simulink model "VITM_sfun"  (R2024b)
settings: Solver=FixedStepDiscrete  StartTime=0.0  StopTime=inf  RelTol=1e-3  EnableMultiTasking=on
values from neighbouring files (symbols this model uses):
  vitc_CellPackVolTol = 12    [VITM_init.m]
  vitc_CellTempFaultTimer = 10    [VITM_init.m]
  vitc_CellTempFilterC = 1.0    (= 1)    [VITM_init.m]
  vitc_CellTempHighFaultReset = 0    [VITM_init.m]
  vitc_CellTempLowFaultReset = 0    [VITM_init.m]
  vitc_CellTempMax = 70    [VITM_init.m]
  vitc_CellTempMin = -40    [VITM_init.m]
  vitc_CellVolFilterC = 1    [VITM_init.m]
  vitc_CellVoltageFaultTimer = 2    [VITM_init.m]
  vitc_CellVoltageHighFaultReset = 0    [VITM_init.m]
  vitc_CellVoltageLowFaultReset = 0    [VITM_init.m]
  vitc_CellVoltageMax = 4.2    [VITM_init.m]
  vitc_CellVoltageMin = 2.7    [VITM_init.m]
  vitc_CoolantInletTFaultReset = 0    [VITM_init.m]
  vitc_CoolantInletTLowerLim = -40    [VITM_init.m]
  vitc_CoolantInletTUpperLim = 70    [VITM_init.m]
  vitc_CoolantOutletTFaultReset = 0    [VITM_init.m]
  vitc_CoolantOutletTLowerLim = -40    [VITM_init.m]
  vitc_CoolantOutletTUpperLim = 70    [VITM_init.m]
  vitc_CoolantTempFaultCounter = 5    [VITM_init.m]
  vitc_CoolantTFilterC = 0.9    [VITM_init.m]
  vitc_HVILFaultCounter = 1    [VITM_init.m]
  vitc_HVILFaultReset = 0    [VITM_init.m]
  vitc_PackCurFilterC = 1    [VITM_init.m]
  vitc_PackCurrentFaultReset = 0    [VITM_init.m]
  vitc_PackCurrentFaultTimer = 1    [VITM_init.m]
  vitc_PackCurrentLimit = 300    [VITM_init.m]
  vitc_PackVolFilterC = 1    [VITM_init.m]
  vitc_PackVoltageFaultReset = 0    [VITM_init.m]
  vitc_PackVoltageFaultTimer = 10    [VITM_init.m]
  vitc_VehVolFilterC = 1    [VITM_init.m]
  vitk_NumberInPara = 1    [VITM_init.m]
  vitk_NumberInSeries = 40    [VITM_init.m]
  vitk_stepSize = 0.1    [VITM_init.m]
settings Model: TunableVars=vitc_CellPackVolTol,vitc_CellTempFaultTimer,vitc_CellTempFilterC,vitc_CellTempHighFaultReset,vitc_CellTempLowFaultReset,vitc_CellTempMax,vitc_CellTempMin,vitc_CellVolFilterC,vitc_CellVoltageFaultTimer,vitc_CellVoltageHighFaultReset,vitc_CellVoltageLowFaultReset,vitc_CellVoltageMax,vitc_CellVoltageMin,vitc_CoolantInletTFaultReset,vitc_CoolantInletTLowerLim,vitc_CoolantInletTUpperLim,vitc_CoolantOutletTFaultReset,vitc_CoolantOutletTLowerLim,vitc_CoolantOutletTUpperLim,vitc_CoolantTFilterC,vitc_CoolantTempFaultCounter,vitc_HVILFaultCounter,vitc_HVILFaultReset,vitc_PackCurFilterC,vitc_PackCurrentFaultReset,vitc_PackCurrentFaultTimer,vitc_PackCurrentLimit,vitc_PackVolFilterC,vitc_PackVoltageFaultReset,vitc_PackVoltageFaultTimer,vitc_VehVolFilterC,vitk_NumberInPara,vitk_NumberInSeries,vitk_stepSize  TunableVarsStorageClass=Auto,Auto,Auto,Auto,Auto,Auto,Auto,Auto,Auto,Auto,Auto,Auto,Auto,Auto,Auto,Auto,Auto,Auto,Auto,Auto,Auto,Auto,Auto,Auto,Auto,Auto,Auto,Auto,Auto,Auto,Auto,Auto,Auto,Auto  TunableVarsTypeQualifier=,,,,,,,,,,,,,,,,,,,,,,,,,,,,,,,,,  Creator=nctzv8  LastModifiedBy=voillat
settings ConfigSet: Description=OpenECU configuration set for code generation under RTW-EC.
settings SolverCC: AlgebraicLoopSolver=TrustRegion  PositivePriorityOrder=on
settings DataIOCC: LimitDataPoints=on  SaveFormat=Array  SignalLoggingSaveFormat=ModelDataLogs
settings OptimizationCC: DefaultParameterBehavior=Inlined  InlineInvariantSignals=on  ExpressionDepthLimit=2147483647  StateBitsets=on  DataBitsets=on  ZeroExternalMemoryAtStartup=off  ZeroInternalMemoryAtStartup=off  NoFixptDivByZeroProtection=on  EfficientFloat2IntCast=on  LifeSpan=1  EfficientTunableParamExpr=on
settings DebuggingCC: SaveWithParameterizedLinksMsg=none  SignalResolutionControl=TryResolveAllWithWarning  MultiTaskDSMMsg=warning  MultiTaskCondExecSysMsg=none  SingleTaskRateTransMsg=error  CheckMatrixSingularityMsg=warning  VectorMatrixConversionMsg=warning  SignalLabelMismatchMsg=warning  UnconnectedInputMsg=warning  UnconnectedOutputMsg=warning  UnconnectedLineMsg=warning  AllowSymbolicDim=off  StateNameClashWarn=warning  SFUnexpectedBacktrackingDiag=warning  SFNoUnconditionalDefaultTransitionDiag=warning  SFExecutionAtInitializationDiag=none  ArithmeticOperatorsInVariantConditions=warning
settings HardwareCC: ProdBitPerPointer=32  ProdBitPerSizeT=32  ProdBitPerPtrDiffT=32  ProdLargestAtomicInteger=Long  ProdLargestAtomicFloat=Double  ProdEndianess=BigEndian  ProdWordSize=32  ProdHWDeviceType=Freescale->32-bit PowerPC  TargetIntDivRoundTo=Zero  TargetEndianess=BigEndian  TargetHWDeviceType=Freescale->32-bit PowerPC  ProdEqTarget=off
settings ModelReferenceCC: EnableRefExpFcnMdlSchedulingChecks=on  PropagateSignalLabelsOutOfModel=off
settings SFSimCC: SimUseLocalCustomCode=off  MATLABDynamicMemAlloc=off  CustomCodeUndefinedFunction=UseInterfaceOnly
settings RTWCC: Description=OpenECU Platform Target (ERT, optimised floating-point code)  SystemTargetFile=openecu_ert.tlc  MakeCommand=make_rtw optimized_floating_point=1  TemplateMakefile=openecu_ert_r2015b_64.tmf  RetainRTWFile=on  RTWUseLocalCustomCode=off  IncludeHyperlinkInReport=on  GPUComputeCapability=3.5
settings CodeAppCC: ForceParamTrailComments=on  IgnoreCustomStorageClasses=off  SimulinkDataObjDesc=on  CustomSymbolStrType=$N$R$M  InsertBlockDesc=on  StateflowObjectComments=on  InternalIdentifier=Classic
settings STFCustomTargetCC: TargetLibSuffix=.a  GenerateSampleERTMain=on  IncludeMdlTerminateFcn=off  CombineOutputUpdateFcns=on  IncludeFileDelimiter=UseQuote  ERTCustomFileBanners=on  SupportContinuousTime=off  RemoveResetFunc=on  MATLABClassNameForMDSCustomization=Simulink.SoftwareTarget.ERTCustomization  SystemTargetFile=openecu_ert.tlc
settings ERTTargetCC: MultiwordLength=2048  GenerateSampleERTMain=on  ParMdlRefBuildCompliant=off  CompOptLevelCompliant=off  ConcurrentExecutionCompliant=off  IncludeMdlTerminateFcn=off  IncludeFileDelimiter=UseQuote  SupportNonInlinedSFcns=on  ModelStepFunctionPrototypeControlCompliant=off  CPPClassGenCompliant=off  UseToolchainInfoCompliant=off  ExtModeMexFile=noextcomm  ERTSrcFileBannerTemplate=oe_code_c_template.cgt  ERTHdrFileBannerTemplate=oe_code_h_template.cgt  ERTDataSrcFileTemplate=oe_data_c_template.cgt  ERTDataHdrFileTemplate=oe_data_h_template.cgt  ERTCustomFileTemplate=example_file_process.tlc  GlobalDataDefinition=InSeparateSourceFile  GlobalDataReference=InSeparateHeaderFile  ConvertIfToSwitch=off  SuppressUnreachableDefaultCases=off  EnableUserReplacementTypes=on  DynamicArrayContainerType=coder::array
settings ConfigComp: CovMetricSettings=dw  CovSaveCumulativeToWorkspaceVar=on  CovSaveSingleToWorkspaceVar=on  CovExternalEMLEnable=off

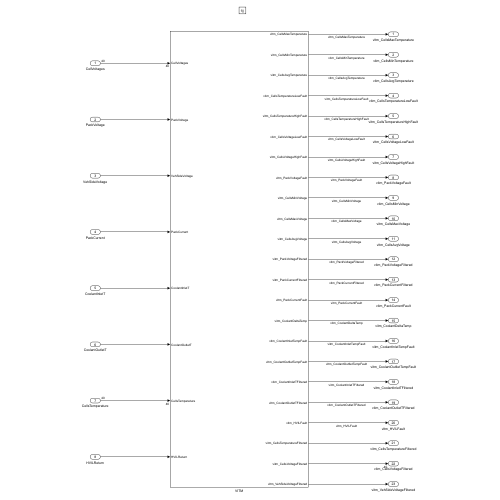
[thumbnail: Simulink's stored preview of the top-level diagram]
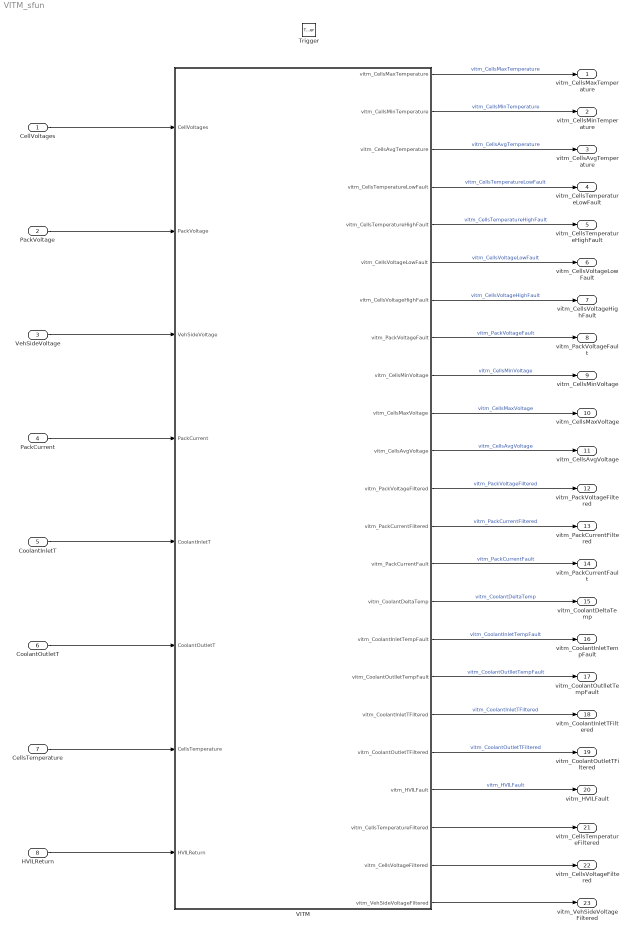
== system VITM_sfun ==
  CellVoltages : Inport  PortDimensions=40
  PackVoltage : Inport  Port=2
  VehSideVoltage : Inport  Port=3
  PackCurrent : Inport  Port=4
  CoolantInletT : Inport  Port=5
  CoolantOutletT : Inport  Port=6
  CellsTemperature : Inport  Port=7  PortDimensions=40
  HVILReturn : Inport  Port=8
  Trigger : TriggerPort  TriggerType=function-call  VariantControl=(inherit)  PortDimensions=1
  VITM : Subsystem  mask{prm_to_disp=[1..10], sfcnParam1=vitc_CellPackVolTol, sfcnParam2=vitc_CellTempFaultTimer, sfcnParam3=vitc_CellTempFilterC, sfcnParam4=vitc_CellTempHighFaultReset, sfcnParam5=vitc_CellTempLowFaultReset, sfcnParam6=vitc_CellTempMax, sfcnParam7=vitc_CellTempMin, sfcnParam8=vitc_CellVolFilterC, sfcnParam9=vitc_CellVoltageFaultTimer, sfcnParam10=vitc_CellVoltageHighFaultReset, sfcnParam11=vitc_CellVoltageLowFaultReset, sfcnParam12=vitc_CellVoltageMax, sfcnParam13=vitc_CellVoltageMin, sfcnParam14=vitc_CoolantInletTFaultReset, sfcnParam15=vitc_CoolantInletTLowerLim, sfcnParam16=vitc_CoolantInletTUpperLim, sfcnParam17=vitc_CoolantOutletTFaultReset, sfcnParam18=vitc_CoolantOutletTLowerLim, sfcnParam19=vitc_CoolantOutletTUpperLim, sfcnParam20=vitc_CoolantTFilterC, sfcnParam21=vitc_CoolantTempFaultCounter, sfcnParam22=vitc_HVILFaultCounter, sfcnParam23=vitc_HVILFaultReset, sfcnParam24=vitc_PackCurFilterC, sfcnParam25=vitc_PackCurrentFaultReset, sfcnParam26=vitc_PackCurrentFaultTimer, sfcnParam27=vitc_PackCurrentLimit, sfcnParam28=vitc_PackVolFilterC, sfcnParam29=vitc_PackVoltageFaultReset, sfcnParam30=vitc_PackVoltageFaultTimer, sfcnParam31=vitc_VehVolFilterC, sfcnParam32=vitk_NumberInPara, sfcnParam33=vitk_NumberInSeries, sfcnParam34=vitk_stepSize}
      mask prompts: prm_to_disp "Display S-function Parameters:"; sfcnParam1 "vitc_CellPackVolTol:"; sfcnParam2 "vitc_CellTempFaultTimer:"; sfcnParam3 "vitc_CellTempFilterC:"; sfcnParam4 "vitc_CellTempHighFaultReset:"; sfcnParam5 "vitc_CellTempLowFaultReset:"; sfcnParam6 "vitc_CellTempMax:"; sfcnParam7 "vitc_CellTempMin:"; sfcnParam8 "vitc_CellVolFilterC:"; sfcnParam9 "vitc_CellVoltageFaultTimer:"; sfcnParam10 "vitc_CellVoltageHighFaultReset:"; sfcnParam11 "vitc_CellVoltageLowFaultReset:"; sfcnParam12 "vitc_CellVoltageMax:"; sfcnParam13 "vitc_CellVoltageMin:"; sfcnParam14 "vitc_CoolantInletTFaultReset:"; sfcnParam15 "vitc_CoolantInletTLowerLim:"; sfcnParam16 "vitc_CoolantInletTUpperLim:"; sfcnParam17 "vitc_CoolantOutletTFaultReset:"; sfcnParam18 "vitc_CoolantOutletTLowerLim:"; sfcnParam19 "vitc_CoolantOutletTUpperLim:"; sfcnParam20 "vitc_CoolantTFilterC:"; sfcnParam21 "vitc_CoolantTempFaultCounter:"; sfcnParam22 "vitc_HVILFaultCounter:"; sfcnParam23 "vitc_HVILFaultReset:"; sfcnParam24 "vitc_PackCurFilterC:"; sfcnParam25 "vitc_PackCurrentFaultReset:"; sfcnParam26 "vitc_PackCurrentFaultTimer:"; sfcnParam27 "vitc_PackCurrentLimit:"; sfcnParam28 "vitc_PackVolFilterC:"; sfcnParam29 "vitc_PackVoltageFaultReset:"; sfcnParam30 "vitc_PackVoltageFaultTimer:"; sfcnParam31 "vitc_VehVolFilterC:"; sfcnParam32 "vitk_NumberInPara:"; sfcnParam33 "vitk_NumberInSeries:"; sfcnParam34 "vitk_stepSize:"
      mask help: Simulink:masks:GenSFuncDesc_MD
      mask Help: eval('feval(''rtwprivate'',''rtwhelpview'',''rtw_sfcn_block'')');
      mask TypeOptions prm_to_disp: [1..10] | [11..20] | [21..30] | [31..34]
      mask Callback prm_to_disp: slmaskprmdispcntrl(gcbh)
  vitm_CellsMaxTemperature : Outport
  vitm_CellsMinTemperature : Outport  Port=2
  vitm_CellsAvgTemperature : Outport  Port=3
  vitm_CellsTemperatureLowFault : Outport  Port=4
  vitm_CellsTemperatureHighFault : Outport  Port=5
  vitm_CellsVoltageLowFault : Outport  Port=6
  vitm_CellsVoltageHighFault : Outport  Port=7
  vitm_PackVoltageFault : Outport  Port=8
  vitm_CellsMinVoltage : Outport  Port=9
  vitm_CellsMaxVoltage : Outport  Port=10
  vitm_CellsAvgVoltage : Outport  Port=11
  vitm_PackVoltageFiltered : Outport  Port=12
  vitm_PackCurrentFiltered : Outport  Port=13
  vitm_PackCurrentFault : Outport  Port=14
  vitm_CoolantDeltaTemp : Outport  Port=15
  vitm_CoolantInletTempFault : Outport  Port=16
  vitm_CoolantOutlletTempFault : Outport  Port=17
  vitm_CoolantInletTFiltered : Outport  Port=18
  vitm_CoolantOutletTFiltered : Outport  Port=19
  vitm_HVILFault : Outport  Port=20
  vitm_CellsTemperatureFiltered : Outport  Port=21
  vitm_CellsVoltageFiltered : Outport  Port=22  PortDimensions=40
  vitm_VehSideVoltageFiltered : Outport  Port=23
  wires:
  CellVoltages/1 -> VITM/1(CellVoltages)
  PackVoltage/1 -> VITM/2(PackVoltage)
  VehSideVoltage/1 -> VITM/3(VehSideVoltage)
  PackCurrent/1 -> VITM/4(PackCurrent)
  CoolantInletT/1 -> VITM/5(CoolantInletT)
  CoolantOutletT/1 -> VITM/6(CoolantOutletT)
  CellsTemperature/1 -> VITM/7(CellsTemperature)
  HVILReturn/1 -> VITM/8(HVILReturn)
  VITM/2(vitm_CellsMinTemperature) -> vitm_CellsMinTemperature/1  "vitm_CellsMinTemperature"
  VITM/3(vitm_CellsAvgTemperature) -> vitm_CellsAvgTemperature/1  "vitm_CellsAvgTemperature"
  VITM/1(vitm_CellsMaxTemperature) -> vitm_CellsMaxTemperature/1  "vitm_CellsMaxTemperature"
  VITM/4(vitm_CellsTemperatureLowFault) -> vitm_CellsTemperatureLowFault/1  "vitm_CellsTemperatureLowFault"
  VITM/6(vitm_CellsVoltageLowFault) -> vitm_CellsVoltageLowFault/1  "vitm_CellsVoltageLowFault"
  VITM/7(vitm_CellsVoltageHighFault) -> vitm_CellsVoltageHighFault/1  "vitm_CellsVoltageHighFault"
  VITM/5(vitm_CellsTemperatureHighFault) -> vitm_CellsTemperatureHighFault/1  "vitm_CellsTemperatureHighFault"
  VITM/9(vitm_CellsMinVoltage) -> vitm_CellsMinVoltage/1  "vitm_CellsMinVoltage"
  VITM/8(vitm_PackVoltageFault) -> vitm_PackVoltageFault/1  "vitm_PackVoltageFault"
  VITM/18(vitm_CoolantInletTFiltered) -> vitm_CoolantInletTFiltered/1  "vitm_CoolantInletTFiltered"
  VITM/10(vitm_CellsMaxVoltage) -> vitm_CellsMaxVoltage/1  "vitm_CellsMaxVoltage"
  VITM/12(vitm_PackVoltageFiltered) -> vitm_PackVoltageFiltered/1  "vitm_PackVoltageFiltered"
  VITM/14(vitm_PackCurrentFault) -> vitm_PackCurrentFault/1  "vitm_PackCurrentFault"
  VITM/15(vitm_CoolantDeltaTemp) -> vitm_CoolantDeltaTemp/1  "vitm_CoolantDeltaTemp"
  VITM/13(vitm_PackCurrentFiltered) -> vitm_PackCurrentFiltered/1  "vitm_PackCurrentFiltered"
  VITM/11(vitm_CellsAvgVoltage) -> vitm_CellsAvgVoltage/1  "vitm_CellsAvgVoltage"
  VITM/16(vitm_CoolantInletTempFault) -> vitm_CoolantInletTempFault/1  "vitm_CoolantInletTempFault"
  VITM/17(vitm_CoolantOutlletTempFault) -> vitm_CoolantOutlletTempFault/1  "vitm_CoolantOutlletTempFault"
  VITM/19(vitm_CoolantOutletTFiltered) -> vitm_CoolantOutletTFiltered/1  "vitm_CoolantOutletTFiltered"
  VITM/23(vitm_VehSideVoltageFiltered) -> vitm_VehSideVoltageFiltered/1
  VITM/22(vitm_CellsVoltageFiltered) -> vitm_CellsVoltageFiltered/1
  VITM/21(vitm_CellsTemperatureFiltered) -> vitm_CellsTemperatureFiltered/1
  VITM/20(vitm_HVILFault) -> vitm_HVILFault/1  "vitm_HVILFault"

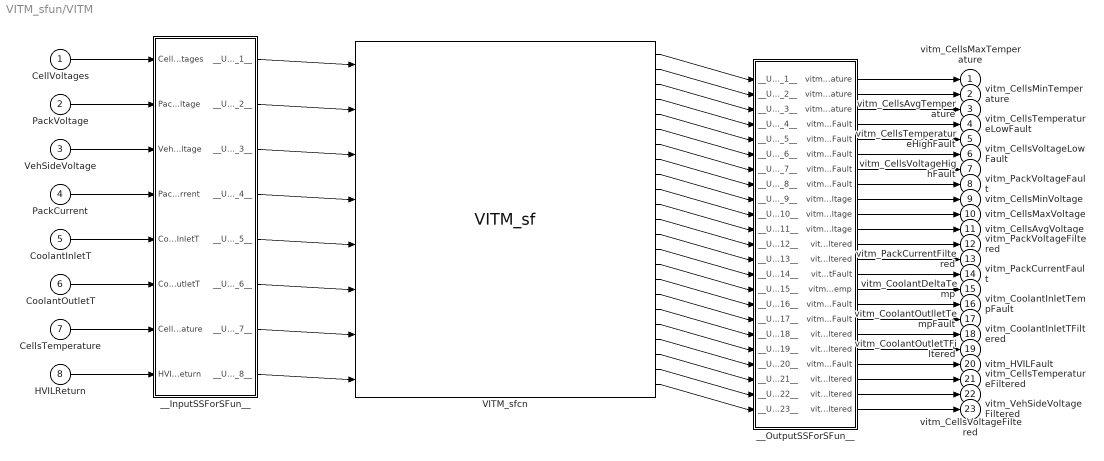
== system VITM_sfun/VITM ==
  CellVoltages : Inport  PortDimensions=40
  PackVoltage : Inport  Port=2
  VehSideVoltage : Inport  Port=3
  PackCurrent : Inport  Port=4
  CoolantInletT : Inport  Port=5
  CoolantOutletT : Inport  Port=6
  CellsTemperature : Inport  Port=7  PortDimensions=40
  HVILReturn : Inport  Port=8
  VITM_sfcn : S-Function  FunctionName=VITM_sf  Parameters=sfcnParam1, sfcnParam2, sfcnParam3, sfcnParam4, sfcnParam5, sfcnParam6, sfcnParam7, sfcnParam8, sfcnParam9, sfcnParam10, sfcnParam11, sfcnParam12, sfcnParam13, sfcnParam14, sfcnParam15, sfcnParam16, sfcnParam17, sfcnParam18, sfcnParam19, sfcnParam20, sfcnParam21, sfcnParam22, sfcnParam23, sfcnParam24, sfcnParam25, sfcnParam26, sfcnParam27, sfcnParam28, sfcnParam29, sfcnParam30, sfcnParam31, sfcnParam32, sfcnParam33, sfcnParam34  SFunctionModules=""  SFunctionDeploymentMode=off  EnableBusSupport=off  mask{rtw_sf_name=VITM_sf, showVar=off, prm_to_disp=[1..10], sfcnParam1=sfcnParam1, sfcnParam2=sfcnParam2, sfcnParam3=sfcnParam3, sfcnParam4=sfcnParam4, sfcnParam5=sfcnParam5, sfcnParam6=sfcnParam6, sfcnParam7=sfcnParam7, sfcnParam8=sfcnParam8, sfcnParam9=sfcnParam9, sfcnParam10=sfcnParam10, sfcnParam11=sfcnParam11, sfcnParam12=sfcnParam12, sfcnParam13=sfcnParam13, sfcnParam14=sfcnParam14, sfcnParam15=sfcnParam15, sfcnParam16=sfcnParam16, sfcnParam17=sfcnParam17, sfcnParam18=sfcnParam18, sfcnParam19=sfcnParam19, sfcnParam20=sfcnParam20, sfcnParam21=sfcnParam21, sfcnParam22=sfcnParam22, sfcnParam23=sfcnParam23, sfcnParam24=sfcnParam24, sfcnParam25=sfcnParam25, sfcnParam26=sfcnParam26, sfcnParam27=sfcnParam27, sfcnParam28=sfcnParam28, sfcnParam29=sfcnParam29, sfcnParam30=sfcnParam30, sfcnParam31=sfcnParam31, sfcnParam32=sfcnParam32, sfcnParam33=sfcnParam33, sfcnParam34=sfcnParam34}
      mask prompts: rtw_sf_name "Simulink:masks:GenSFuncName_MP"; showVar "Simulink:masks:GenSFuncShowModuleList_MP"; prm_to_disp "Display S-function Parameters:"; sfcnParam1 "vitc_CellPackVolTol:"; sfcnParam2 "vitc_CellTempFaultTimer:"; sfcnParam3 "vitc_CellTempFilterC:"; sfcnParam4 "vitc_CellTempHighFaultReset:"; sfcnParam5 "vitc_CellTempLowFaultReset:"; sfcnParam6 "vitc_CellTempMax:"; sfcnParam7 "vitc_CellTempMin:"; sfcnParam8 "vitc_CellVolFilterC:"; sfcnParam9 "vitc_CellVoltageFaultTimer:"; sfcnParam10 "vitc_CellVoltageHighFaultReset:"; sfcnParam11 "vitc_CellVoltageLowFaultReset:"; sfcnParam12 "vitc_CellVoltageMax:"; sfcnParam13 "vitc_CellVoltageMin:"; sfcnParam14 "vitc_CoolantInletTFaultReset:"; sfcnParam15 "vitc_CoolantInletTLowerLim:"; sfcnParam16 "vitc_CoolantInletTUpperLim:"; sfcnParam17 "vitc_CoolantOutletTFaultReset:"; sfcnParam18 "vitc_CoolantOutletTLowerLim:"; sfcnParam19 "vitc_CoolantOutletTUpperLim:"; sfcnParam20 "vitc_CoolantTFilterC:"; sfcnParam21 "vitc_CoolantTempFaultCounter:"; sfcnParam22 "vitc_HVILFaultCounter:"; sfcnParam23 "vitc_HVILFaultReset:"; sfcnParam24 "vitc_PackCurFilterC:"; sfcnParam25 "vitc_PackCurrentFaultReset:"; sfcnParam26 "vitc_PackCurrentFaultTimer:"; sfcnParam27 "vitc_PackCurrentLimit:"; sfcnParam28 "vitc_PackVolFilterC:"; sfcnParam29 "vitc_PackVoltageFaultReset:"; sfcnParam30 "vitc_PackVoltageFaultTimer:"; sfcnParam31 "vitc_VehVolFilterC:"; sfcnParam32 "vitk_NumberInPara:"; sfcnParam33 "vitk_NumberInSeries:"; sfcnParam34 "vitk_stepSize:"
      mask help: Simulink:masks:GenSFuncDesc_MD
      mask init:
      | displist = '';
      | if ~strcmp(get_param(gcb, 'FunctionName'), rtw_sf_name);
      |   set_param(gcb, 'FunctionName', rtw_sf_name);
      | end
      | % Check if we are generating code
      | rtw_mode = false;
      | if strcmpi(get_param(bdroot(gcb),'SimulationStatus'),'Initializing')
      | 	rtw_mode = strcmpi(get_param(bdroot(gcb),'BuildingRTWCode'),'on') && ...
      | 		~strcmpi(get_param(bdroot(gcb),'TargetStyle'),'SimulationTarget');
      | end
      | if showVar || rtw_mode
      | 	if exist('rtwsfunc') == 2 | exist('rtwsfunc') == 6
      | 		tmplist = rtwsfunc(rtw_sf_name,gcb);
      | 		tmplist = DAStudio.message('Simulink:masks:GenSFuncListOfModules_IC', tmplist);
      | 	elseif showVar
      | 		tmplist1 = DAStudio.message('Simulink:masks:GenSFuncListOfModules_IC', '');
      |         tmplist2 = DAStudio.message('Simulink:masks:GenSFuncNotLicensed_IC');
      |         tmplist = [tmplist1 tmplist2];
      |  	end
      | end
      | if showVar
      |   displist = tmplist;
      | end
      settings: CopyFcn=|
      | if ~strcmp(get_param(gcb,'Linkstatus'),'none') && ...
      | ~strcmp(get_param(gcb,'Linkstatus'),'implicit')
      |   set_param(gcb,'LinkStatus','none');
      | end
      mask Help: eval('feval(''rtwprivate'',''rtwhelpview'',''rtw_sfcn_block'')');
      mask TypeOptions prm_to_disp: [1..10] | [11..20] | [21..30] | [31..34]
      mask Callback prm_to_disp: slmaskprmdispcntrl(gcbh)
      mask Display:
      | port_label('input',1,'CellVoltages');
      | port_label('input',2,'PackVoltage');
      | port_label('input',3,'VehSideVoltage');
      | port_label('input',4,'PackCurrent');
      | port_label('input',5,'CoolantInletT');
      | port_label('input',6,'CoolantOutletT');
      | port_label('input',7,'CellsTemperature');
      | port_label('input',8,'HVILReturn');
      | port_label('output',1,'vitm_CellsMaxTemperature');
      | port_label('output',2,'vitm_CellsMinTemperature');
      | port_label('output',3,'vitm_CellsAvgTemperature');
      | port_label('output',4,'vitm_CellsTemperatureLowFault');
      | port_label('output',5,'vitm_CellsTemperatureHighFault');
      | port_label('output',6,'vitm_CellsVoltageLowFault');
      | port_label('output',7,'vitm_CellsVoltageHighFault');
      | port_label('output',8,'vitm_PackVoltageFault');
      | port_label('output',9,'vitm_CellsMinVoltage');
      | port_label('output',10,'vitm_CellsMaxVoltage');
      | port_label('output',11,'vitm_CellsAvgVoltage');
      | port_label('output',12,'vitm_PackVoltageFiltered');
      | port_label('output',13,'vitm_PackCurrentFiltered');
      | port_label('output',14,'vitm_PackCurrentFault');
      | port_label('output',15,'vitm_CoolantDeltaTemp');
      | port_label('output',16,'vitm_CoolantInletTempFault');
      | port_label('output',17,'vitm_CoolantOutlletTempFault');
      | port_label('output',18,'vitm_CoolantInletTFiltered');
      | port_label('output',19,'vitm_CoolantOutletTFiltered');
      | port_label('output',20,'vitm_HVILFault');
      | port_label('output',21,'vitm_CellsTemperatureFiltered');
      | port_label('output',22,'vitm_CellsVoltageFiltered');
      | port_label('output',23,'vitm_VehSideVoltageFiltered');
  __InputSSForSFun__ : Subsystem
  __OutputSSForSFun__ : Subsystem
  vitm_CellsMaxTemperature : Outport
  vitm_CellsMinTemperature : Outport  Port=2
  vitm_CellsAvgTemperature : Outport  Port=3
  vitm_CellsTemperatureLowFault : Outport  Port=4
  vitm_CellsTemperatureHighFault : Outport  Port=5
  vitm_CellsVoltageLowFault : Outport  Port=6
  vitm_CellsVoltageHighFault : Outport  Port=7
  vitm_PackVoltageFault : Outport  Port=8
  vitm_CellsMinVoltage : Outport  Port=9
  vitm_CellsMaxVoltage : Outport  Port=10
  vitm_CellsAvgVoltage : Outport  Port=11
  vitm_PackVoltageFiltered : Outport  Port=12
  vitm_PackCurrentFiltered : Outport  Port=13
  vitm_PackCurrentFault : Outport  Port=14
  vitm_CoolantDeltaTemp : Outport  Port=15
  vitm_CoolantInletTempFault : Outport  Port=16
  vitm_CoolantOutlletTempFault : Outport  Port=17
  vitm_CoolantInletTFiltered : Outport  Port=18
  vitm_CoolantOutletTFiltered : Outport  Port=19
  vitm_HVILFault : Outport  Port=20
  vitm_CellsTemperatureFiltered : Outport  Port=21
  vitm_CellsVoltageFiltered : Outport  Port=22
  vitm_VehSideVoltageFiltered : Outport  Port=23
  wires:
  CellVoltages/1 -> __InputSSForSFun__/1(CellVoltages)
  PackVoltage/1 -> __InputSSForSFun__/2(PackVoltage)
  VehSideVoltage/1 -> __InputSSForSFun__/3(VehSideVoltage)
  PackCurrent/1 -> __InputSSForSFun__/4(PackCurrent)
  CoolantInletT/1 -> __InputSSForSFun__/5(CoolantInletT)
  CoolantOutletT/1 -> __InputSSForSFun__/6(CoolantOutletT)
  CellsTemperature/1 -> __InputSSForSFun__/7(CellsTemperature)
  HVILReturn/1 -> __InputSSForSFun__/8(HVILReturn)
  __InputSSForSFun__/1(__UniqueOutportName__1__) -> VITM_sfcn/1
  __InputSSForSFun__/2(__UniqueOutportName__2__) -> VITM_sfcn/2
  __InputSSForSFun__/3(__UniqueOutportName__3__) -> VITM_sfcn/3
  __InputSSForSFun__/4(__UniqueOutportName__4__) -> VITM_sfcn/4
  __InputSSForSFun__/5(__UniqueOutportName__5__) -> VITM_sfcn/5
  __InputSSForSFun__/6(__UniqueOutportName__6__) -> VITM_sfcn/6
  __InputSSForSFun__/7(__UniqueOutportName__7__) -> VITM_sfcn/7
  __InputSSForSFun__/8(__UniqueOutportName__8__) -> VITM_sfcn/8
  VITM_sfcn/1 -> __OutputSSForSFun__/1(__UniqueInportName__1__)
  VITM_sfcn/2 -> __OutputSSForSFun__/2(__UniqueInportName__2__)
  VITM_sfcn/3 -> __OutputSSForSFun__/3(__UniqueInportName__3__)
  VITM_sfcn/4 -> __OutputSSForSFun__/4(__UniqueInportName__4__)
  VITM_sfcn/5 -> __OutputSSForSFun__/5(__UniqueInportName__5__)
  VITM_sfcn/6 -> __OutputSSForSFun__/6(__UniqueInportName__6__)
  VITM_sfcn/7 -> __OutputSSForSFun__/7(__UniqueInportName__7__)
  VITM_sfcn/8 -> __OutputSSForSFun__/8(__UniqueInportName__8__)
  VITM_sfcn/9 -> __OutputSSForSFun__/9(__UniqueInportName__9__)
  VITM_sfcn/10 -> __OutputSSForSFun__/10(__UniqueInportName__10__)
  VITM_sfcn/11 -> __OutputSSForSFun__/11(__UniqueInportName__11__)
  VITM_sfcn/12 -> __OutputSSForSFun__/12(__UniqueInportName__12__)
  VITM_sfcn/13 -> __OutputSSForSFun__/13(__UniqueInportName__13__)
  VITM_sfcn/14 -> __OutputSSForSFun__/14(__UniqueInportName__14__)
  VITM_sfcn/15 -> __OutputSSForSFun__/15(__UniqueInportName__15__)
  VITM_sfcn/16 -> __OutputSSForSFun__/16(__UniqueInportName__16__)
  VITM_sfcn/17 -> __OutputSSForSFun__/17(__UniqueInportName__17__)
  VITM_sfcn/18 -> __OutputSSForSFun__/18(__UniqueInportName__18__)
  VITM_sfcn/19 -> __OutputSSForSFun__/19(__UniqueInportName__19__)
  VITM_sfcn/20 -> __OutputSSForSFun__/20(__UniqueInportName__20__)
  VITM_sfcn/21 -> __OutputSSForSFun__/21(__UniqueInportName__21__)
  VITM_sfcn/22 -> __OutputSSForSFun__/22(__UniqueInportName__22__)
  VITM_sfcn/23 -> __OutputSSForSFun__/23(__UniqueInportName__23__)
  __OutputSSForSFun__/1(vitm_CellsMaxTemperature) -> vitm_CellsMaxTemperature/1
  __OutputSSForSFun__/2(vitm_CellsMinTemperature) -> vitm_CellsMinTemperature/1
  __OutputSSForSFun__/3(vitm_CellsAvgTemperature) -> vitm_CellsAvgTemperature/1
  __OutputSSForSFun__/4(vitm_CellsTemperatureLowFault) -> vitm_CellsTemperatureLowFault/1
  __OutputSSForSFun__/5(vitm_CellsTemperatureHighFault) -> vitm_CellsTemperatureHighFault/1
  __OutputSSForSFun__/6(vitm_CellsVoltageLowFault) -> vitm_CellsVoltageLowFault/1
  __OutputSSForSFun__/7(vitm_CellsVoltageHighFault) -> vitm_CellsVoltageHighFault/1
  __OutputSSForSFun__/8(vitm_PackVoltageFault) -> vitm_PackVoltageFault/1
  __OutputSSForSFun__/9(vitm_CellsMinVoltage) -> vitm_CellsMinVoltage/1
  __OutputSSForSFun__/10(vitm_CellsMaxVoltage) -> vitm_CellsMaxVoltage/1
  __OutputSSForSFun__/11(vitm_CellsAvgVoltage) -> vitm_CellsAvgVoltage/1
  __OutputSSForSFun__/12(vitm_PackVoltageFiltered) -> vitm_PackVoltageFiltered/1
  __OutputSSForSFun__/13(vitm_PackCurrentFiltered) -> vitm_PackCurrentFiltered/1
  __OutputSSForSFun__/14(vitm_PackCurrentFault) -> vitm_PackCurrentFault/1
  __OutputSSForSFun__/15(vitm_CoolantDeltaTemp) -> vitm_CoolantDeltaTemp/1
  __OutputSSForSFun__/16(vitm_CoolantInletTempFault) -> vitm_CoolantInletTempFault/1
  __OutputSSForSFun__/17(vitm_CoolantOutlletTempFault) -> vitm_CoolantOutlletTempFault/1
  __OutputSSForSFun__/18(vitm_CoolantInletTFiltered) -> vitm_CoolantInletTFiltered/1
  __OutputSSForSFun__/19(vitm_CoolantOutletTFiltered) -> vitm_CoolantOutletTFiltered/1
  __OutputSSForSFun__/20(vitm_HVILFault) -> vitm_HVILFault/1
  __OutputSSForSFun__/21(vitm_CellsTemperatureFiltered) -> vitm_CellsTemperatureFiltered/1
  __OutputSSForSFun__/22(vitm_CellsVoltageFiltered) -> vitm_CellsVoltageFiltered/1
  __OutputSSForSFun__/23(vitm_VehSideVoltageFiltered) -> vitm_VehSideVoltageFiltered/1

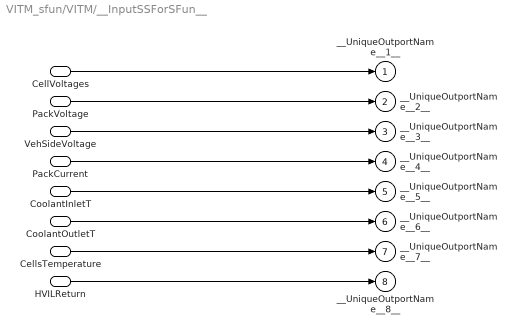
== system VITM_sfun/VITM/__InputSSForSFun__ ==
  CellVoltages : Inport  PortDimensions=40
  PackVoltage : Inport  Port=2
  VehSideVoltage : Inport  Port=3
  PackCurrent : Inport  Port=4
  CoolantInletT : Inport  Port=5
  CoolantOutletT : Inport  Port=6
  CellsTemperature : Inport  Port=7  PortDimensions=40
  HVILReturn : Inport  Port=8
  __UniqueOutportName__1__ : Outport
  __UniqueOutportName__2__ : Outport  Port=2
  __UniqueOutportName__3__ : Outport  Port=3
  __UniqueOutportName__4__ : Outport  Port=4
  __UniqueOutportName__5__ : Outport  Port=5
  __UniqueOutportName__6__ : Outport  Port=6
  __UniqueOutportName__7__ : Outport  Port=7
  __UniqueOutportName__8__ : Outport  Port=8
  wires:
  CellVoltages/1 -> __UniqueOutportName__1__/1
  PackVoltage/1 -> __UniqueOutportName__2__/1
  VehSideVoltage/1 -> __UniqueOutportName__3__/1
  PackCurrent/1 -> __UniqueOutportName__4__/1
  CoolantInletT/1 -> __UniqueOutportName__5__/1
  CoolantOutletT/1 -> __UniqueOutportName__6__/1
  CellsTemperature/1 -> __UniqueOutportName__7__/1
  HVILReturn/1 -> __UniqueOutportName__8__/1

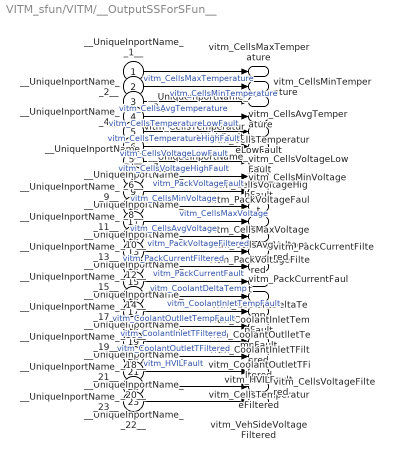
== system VITM_sfun/VITM/__OutputSSForSFun__ ==
  __UniqueInportName__1__ : Inport
  __UniqueInportName__2__ : Inport  Port=2
  __UniqueInportName__3__ : Inport  Port=3
  __UniqueInportName__4__ : Inport  Port=4
  __UniqueInportName__5__ : Inport  Port=5
  __UniqueInportName__6__ : Inport  Port=6
  __UniqueInportName__7__ : Inport  Port=7
  __UniqueInportName__8__ : Inport  Port=8
  __UniqueInportName__9__ : Inport  Port=9
  __UniqueInportName__10__ : Inport  Port=10
  __UniqueInportName__11__ : Inport  Port=11
  __UniqueInportName__12__ : Inport  Port=12
  __UniqueInportName__13__ : Inport  Port=13
  __UniqueInportName__14__ : Inport  Port=14
  __UniqueInportName__15__ : Inport  Port=15
  __UniqueInportName__16__ : Inport  Port=16
  __UniqueInportName__17__ : Inport  Port=17
  __UniqueInportName__18__ : Inport  Port=18
  __UniqueInportName__19__ : Inport  Port=19
  __UniqueInportName__20__ : Inport  Port=20
  __UniqueInportName__21__ : Inport  Port=21
  __UniqueInportName__22__ : Inport  Port=22
  __UniqueInportName__23__ : Inport  Port=23
  vitm_CellsMaxTemperature : Outport
  vitm_CellsMinTemperature : Outport  Port=2
  vitm_CellsAvgTemperature : Outport  Port=3
  vitm_CellsTemperatureLowFault : Outport  Port=4
  vitm_CellsTemperatureHighFault : Outport  Port=5
  vitm_CellsVoltageLowFault : Outport  Port=6
  vitm_CellsVoltageHighFault : Outport  Port=7
  vitm_PackVoltageFault : Outport  Port=8
  vitm_CellsMinVoltage : Outport  Port=9
  vitm_CellsMaxVoltage : Outport  Port=10
  vitm_CellsAvgVoltage : Outport  Port=11
  vitm_PackVoltageFiltered : Outport  Port=12
  vitm_PackCurrentFiltered : Outport  Port=13
  vitm_PackCurrentFault : Outport  Port=14
  vitm_CoolantDeltaTemp : Outport  Port=15
  vitm_CoolantInletTempFault : Outport  Port=16
  vitm_CoolantOutlletTempFault : Outport  Port=17
  vitm_CoolantInletTFiltered : Outport  Port=18
  vitm_CoolantOutletTFiltered : Outport  Port=19
  vitm_HVILFault : Outport  Port=20
  vitm_CellsTemperatureFiltered : Outport  Port=21
  vitm_CellsVoltageFiltered : Outport  Port=22
  vitm_VehSideVoltageFiltered : Outport  Port=23
  wires:
  __UniqueInportName__1__/1 -> vitm_CellsMaxTemperature/1  "vitm_CellsMaxTemperature"
  __UniqueInportName__2__/1 -> vitm_CellsMinTemperature/1  "vitm_CellsMinTemperature"
  __UniqueInportName__3__/1 -> vitm_CellsAvgTemperature/1  "vitm_CellsAvgTemperature"
  __UniqueInportName__4__/1 -> vitm_CellsTemperatureLowFault/1  "vitm_CellsTemperatureLowFault"
  __UniqueInportName__5__/1 -> vitm_CellsTemperatureHighFault/1  "vitm_CellsTemperatureHighFault"
  __UniqueInportName__6__/1 -> vitm_CellsVoltageLowFault/1  "vitm_CellsVoltageLowFault"
  __UniqueInportName__7__/1 -> vitm_CellsVoltageHighFault/1  "vitm_CellsVoltageHighFault"
  __UniqueInportName__8__/1 -> vitm_PackVoltageFault/1  "vitm_PackVoltageFault"
  __UniqueInportName__9__/1 -> vitm_CellsMinVoltage/1  "vitm_CellsMinVoltage"
  __UniqueInportName__10__/1 -> vitm_CellsMaxVoltage/1  "vitm_CellsMaxVoltage"
  __UniqueInportName__11__/1 -> vitm_CellsAvgVoltage/1  "vitm_CellsAvgVoltage"
  __UniqueInportName__12__/1 -> vitm_PackVoltageFiltered/1  "vitm_PackVoltageFiltered"
  __UniqueInportName__13__/1 -> vitm_PackCurrentFiltered/1  "vitm_PackCurrentFiltered"
  __UniqueInportName__14__/1 -> vitm_PackCurrentFault/1  "vitm_PackCurrentFault"
  __UniqueInportName__15__/1 -> vitm_CoolantDeltaTemp/1  "vitm_CoolantDeltaTemp"
  __UniqueInportName__16__/1 -> vitm_CoolantInletTempFault/1  "vitm_CoolantInletTempFault"
  __UniqueInportName__17__/1 -> vitm_CoolantOutlletTempFault/1  "vitm_CoolantOutlletTempFault"
  __UniqueInportName__18__/1 -> vitm_CoolantInletTFiltered/1  "vitm_CoolantInletTFiltered"
  __UniqueInportName__19__/1 -> vitm_CoolantOutletTFiltered/1  "vitm_CoolantOutletTFiltered"
  __UniqueInportName__20__/1 -> vitm_HVILFault/1  "vitm_HVILFault"
  __UniqueInportName__21__/1 -> vitm_CellsTemperatureFiltered/1
  __UniqueInportName__22__/1 -> vitm_CellsVoltageFiltered/1
  __UniqueInportName__23__/1 -> vitm_VehSideVoltageFiltered/1
